simulink model "decomposition"  (Simulink 7.6)
settings: Solver=ode45  StartTime=0.0  StopTime=10.0  MaxStep=1e-2  RelTol=1e-3
libraries: simulink x4
settings Model: Creator=John  LastModifiedBy=John
settings DebuggingCC: SolverPrmCheckMsg=none

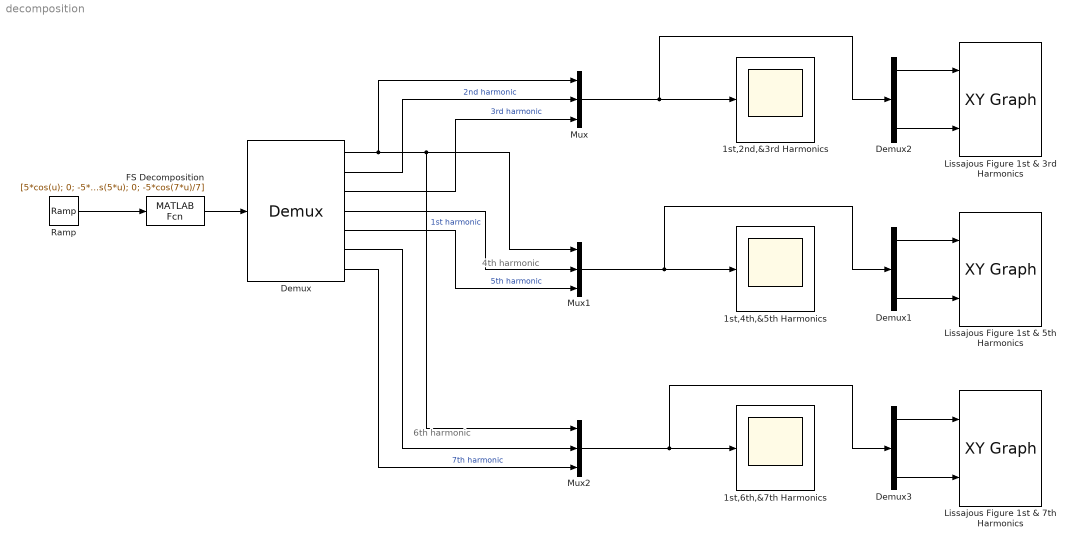
== system decomposition ==
  note: 4th harmonic
  note: 6th harmonic
  1st,2nd,&3rd Harmonics : Scope
  1st,4th,&5th Harmonics : Scope
  1st,6th,&7th Harmonics : Scope
      settings: SaveName=ScopeData2
  Demux : Demux  Description=|  Outputs=7
      | k=1
      | k=2
      | k=3
  Demux1 : Demux  Outputs=3
  Demux2 : Demux  Outputs=3
  Demux3 : Demux  Outputs=3
  FS Decomposition : MATLABFcn  MATLABFcn=[5*cos(u); 0; -5*cos(3*u)/3; 0; cos(5*u); 0; -5*cos(7*u)/7]  OutputDimensions=7
  Lissajous Figure 1st & 3rd Harmonics : simulink/Sinks/XY Graph  SystemSampleTime=-1  xmin=-5  xmax=5  ymin=-5  ymax=5  st=-1
  Lissajous Figure 1st & 5th Harmonics : simulink/Sinks/XY Graph  SystemSampleTime=-1  xmin=-5  xmax=5  ymin=-5  ymax=5  st=-1
  Lissajous Figure 1st & 7th Harmonics : simulink/Sinks/XY Graph  SystemSampleTime=-1  xmin=-5  xmax=5  ymin=-5  ymax=5  st=-1
  Mux : Mux  Inputs=3
  Mux1 : Mux  Inputs=3
  Mux2 : Mux  Inputs=3
  Ramp : simulink/Sources/Ramp  SystemSampleTime=-1  slope=pi  start=0  X0=0
  wires:
  Ramp/1 -> FS Decomposition/1
  FS Decomposition/1 -> Demux/1
  Demux/1 -> Mux/1, Mux1/1, Mux2/1  "1st harmonic"
  Demux/2 -> Mux/2  "2nd harmonic"
  Demux/3 -> Mux/3  "3rd harmonic"
  Demux/4 -> Mux1/2
  Demux/5 -> Mux1/3  "5th harmonic"
  Demux/6 -> Mux2/2
  Demux/7 -> Mux2/3  "7th harmonic"
  Mux/1 -> 1st,2nd,&3rd Harmonics/1, Demux2/1
  Mux1/1 -> 1st,4th,&5th Harmonics/1, Demux1/1
  Mux2/1 -> 1st,6th,&7th Harmonics/1, Demux3/1
  Demux2/1 -> Lissajous Figure 1st & 3rd Harmonics/1
  Demux2/3 -> Lissajous Figure 1st & 3rd Harmonics/2
  Demux1/1 -> Lissajous Figure 1st & 5th Harmonics/1
  Demux1/3 -> Lissajous Figure 1st & 5th Harmonics/2
  Demux3/1 -> Lissajous Figure 1st & 7th Harmonics/1
  Demux3/3 -> Lissajous Figure 1st & 7th Harmonics/2
